simulink model "cw7_3_3"  (R2019a)
settings: Solver=VariableStepAuto  StartTime=0.0  StopTime=50  RelTol=1e-10  EnableMultiTasking=on
values from neighbouring files (symbols this model uses):
  k1 = 2    [SchematyBlokowe.m]    (also in TIPS_Lab_6_Zad_Dom.m = 0:N1-1)
  k2 = 2    [SchematyBlokowe.m]    (also in TIPS_Lab_6_Zad_Dom.m = 0:N2-1)
  kp = 5    [AutomatykaCw5.m]    (also in SchematyBlokowe.m = 2)
  kp1 = 0.3125    [SchematyBlokowe.m]
  kp2 = 0.2    [SchematyBlokowe.m]
  kp3 = 10    [SchematyBlokowe.m]
  T11 = 4    [SchematyBlokowe.m]
  T12 = 5    [SchematyBlokowe.m]
  T21 = 5    [SchematyBlokowe.m]
  T22 = 5    [SchematyBlokowe.m]
  Ti = 1    [SchematyBlokowe.m]
  Ti1 = 5    [SchematyBlokowe.m]
  Ti2 = 4    [SchematyBlokowe.m]
  Ti3 = 30    [SchematyBlokowe.m]
libraries: simulink x1
settings Model: Creator=Pawel  LastModifiedBy=ASUS_PEPE
settings DataIOCC: LimitDataPoints=on  ReturnWorkspaceOutputs=off
settings OptimizationCC: LifeSpan=inf
settings DebuggingCC: AllowSymbolicDim=off  SFUnexpectedBacktrackingDiag=warning  SFNoUnconditionalDefaultTransitionDiag=warning  SFExecutionAtInitializationDiag=none  ArithmeticOperatorsInVariantConditions=warning
settings ModelReferenceCC: PropagateSignalLabelsOutOfModel=off
settings SFSimCC: SimUseLocalCustomCode=off
settings RTWCC: RTWUseLocalCustomCode=off
settings CodeAppCC: StateflowObjectComments=on
settings GRTTargetCC: TargetLangStandard=C89/C90 (ANSI)
settings ConfigComp: CovMetricSettings=dw  CovHtmlReporting=on  CovSaveCumulativeToWorkspaceVar=on  CovSaveSingleToWorkspaceVar=on  CovExternalEMLEnable=off

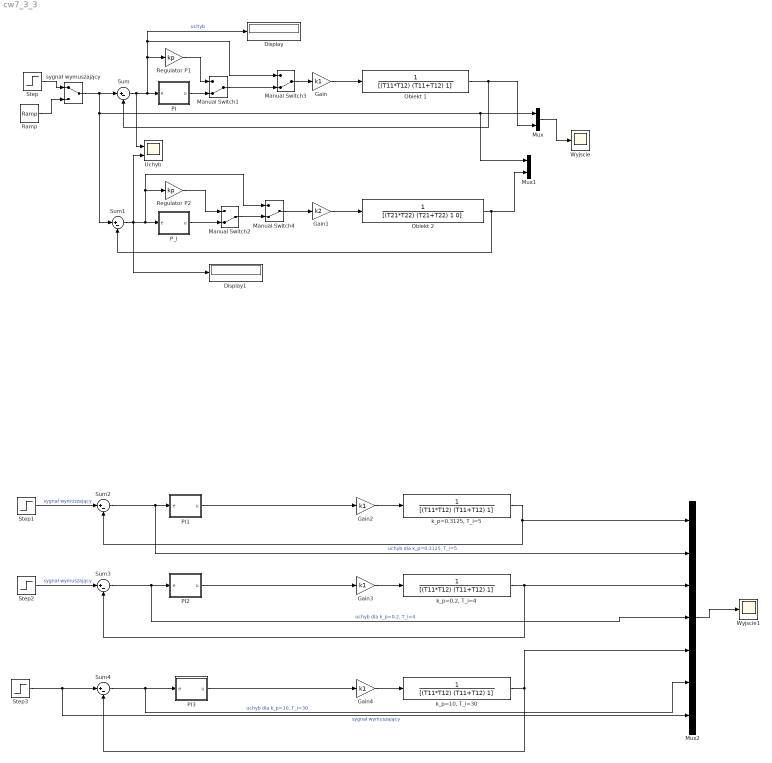
== system cw7_3_3 ==
  Display : Display
  Display1 : Display
  Gain{,2..4} (4 alike) : Gain  Gain=k1
  Gain1 : Gain  Gain=k2
  Manual Switch{1..4} (4 alike) : ManualSwitch  CurrentSetting=0
  Mux : Mux  Inputs=2
  Mux1 : Mux  Inputs=2
  Mux2 : Mux  Inputs=7
  Obiekt 1 : TransferFcn  Numerator=1  Denominator=[(T11*T12) (T11+T12) 1]
  Obiekt 2 : TransferFcn  Numerator=1  Denominator=[(T21*T22) (T21+T22) 1 0]
  PI : Subsystem
  "PI1 " : Subsystem
  PI2 : Subsystem
  PI3 : Subsystem
  P_I : Subsystem
  Ramp : simulink/Sources/Ramp  slope=1  start=0  InitialOutput=0
  Regulator P1 : Gain  Gain=kp
  Regulator P2 : Gain  Gain=kp
  Step : Step  SampleTime=0
  Step1 : Step  Before=1  SampleTime=0
  Step2 : Step  Before=1  SampleTime=0
  Step3 : Step  Before=1  SampleTime=0
  Sum{,1..4} (5 alike) : Sum  Inputs=|+-
  Uchyb : Scope  NumInputPorts=2
  Wyjscie : Scope
  Wyjscie1 : Scope
  "k_p=0.2, T_i=4" : TransferFcn  Numerator=1  Denominator=[(T11*T12) (T11+T12) 1]
  "k_p=0.3125, T_i=5" : TransferFcn  Numerator=1  Denominator=[(T11*T12) (T11+T12) 1]
  "k_p=10, T_i=30" : TransferFcn  Numerator=1  Denominator=[(T11*T12) (T11+T12) 1]
  sygnał wymuszający : ManualSwitch
  wires:
  Obiekt 1/1 -> Sum/2, Mux/2
  Sum/1 -> Manual Switch3/1, Display/1, Regulator P1/1, PI/1(e), Uchyb/1  "uchyb"
  Obiekt 2/1 -> Sum1/2, Mux1/2
  Sum1/1 -> Display1/1, Uchyb/2, Manual Switch4/1, Regulator P2/1, P_I/1(e)
  Gain/1 -> Obiekt 1/1
  Gain1/1 -> Obiekt 2/1
  sygnał wymuszający/1 -> Sum1/1, Mux1/1, Mux/1, Sum/1
  Step/1 -> sygnał wymuszający/1
  Ramp/1 -> sygnał wymuszający/2
  Manual Switch1/1 -> Manual Switch3/2
  PI/1(u) -> Manual Switch1/2
  Regulator P1/1 -> Manual Switch1/1
  Regulator P2/1 -> Manual Switch2/1
  P_I/1(u) -> Manual Switch2/2
  Manual Switch2/1 -> Manual Switch4/2
  Manual Switch3/1 -> Gain/1
  Manual Switch4/1 -> Gain1/1
  Mux/1 -> Wyjscie/1
  Step1/1 -> Sum2/1  "sygnał wymuszający"
  Gain2/1 -> "k_p=0.3125, T_i=5"/1
  "k_p=0.3125, T_i=5"/1 -> Sum2/2, Mux2/1
  PI3/1(u) -> Gain4/1
  PI2/1(u) -> Gain3/1
  "PI1 "/1(u) -> Gain2/1
  Sum2/1 -> Mux2/2, "PI1 "/1(e)  "uchyb dla k_p=0.3125, T_i=5"
  Gain4/1 -> "k_p=10, T_i=30"/1
  Gain3/1 -> "k_p=0.2, T_i=4"/1
  Sum3/1 -> Mux2/4, PI2/1(e)  "uchyb dla k_p=0.2, T_i=4"
  Step2/1 -> Sum3/1  "sygnał wymuszający"
  Sum4/1 -> Mux2/6, PI3/1(e)  "uchyb dla k_p=10, T_i=30"
  Step3/1 -> Mux2/7, Sum4/1  "sygnał wymuszający"
  "k_p=0.2, T_i=4"/1 -> Mux2/3, Sum3/2
  Mux2/1 -> Wyjscie1/1
  "k_p=10, T_i=30"/1 -> Mux2/5, Sum4/2

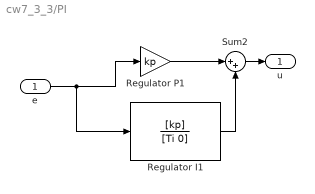
== system cw7_3_3/PI ==
  e : Inport
  Regulator I1 : TransferFcn  Numerator=[kp]  Denominator=[Ti 0]
  Regulator P1 : Gain  Gain=kp
  Sum2 : Sum  Inputs=|++
  u : Outport
  wires:
  Regulator I1/1 -> Sum2/2
  Sum2/1 -> u/1
  e/1 -> Regulator I1/1, Regulator P1/1
  Regulator P1/1 -> Sum2/1

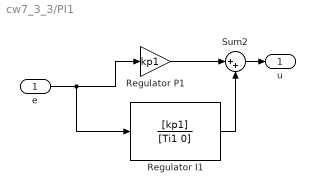
== system cw7_3_3/PI1  ==
  e : Inport
  Regulator I1 : TransferFcn  Numerator=[kp1]  Denominator=[Ti1 0]
  Regulator P1 : Gain  Gain=kp1
  Sum2 : Sum  Inputs=|++
  u : Outport
  wires:
  Regulator I1/1 -> Sum2/2
  Sum2/1 -> u/1
  e/1 -> Regulator I1/1, Regulator P1/1
  Regulator P1/1 -> Sum2/1

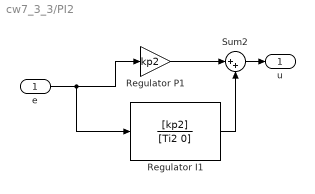
== system cw7_3_3/PI2 ==
  e : Inport
  Regulator I1 : TransferFcn  Numerator=[kp2]  Denominator=[Ti2 0]
  Regulator P1 : Gain  Gain=kp2
  Sum2 : Sum  Inputs=|++
  u : Outport
  wires:
  Regulator I1/1 -> Sum2/2
  Sum2/1 -> u/1
  e/1 -> Regulator I1/1, Regulator P1/1
  Regulator P1/1 -> Sum2/1

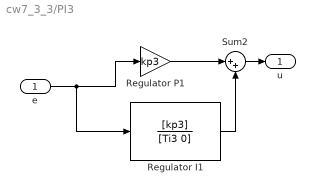
== system cw7_3_3/PI3 ==
  e : Inport
  Regulator I1 : TransferFcn  Numerator=[kp3]  Denominator=[Ti3 0]
  Regulator P1 : Gain  Gain=kp3
  Sum2 : Sum  Inputs=|++
  u : Outport
  wires:
  Regulator I1/1 -> Sum2/2
  Sum2/1 -> u/1
  e/1 -> Regulator I1/1, Regulator P1/1
  Regulator P1/1 -> Sum2/1

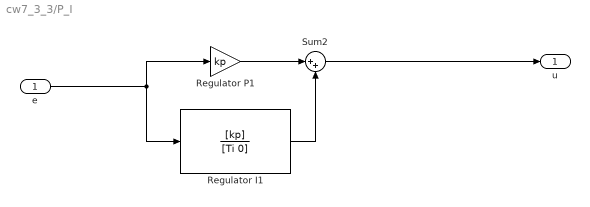
== system cw7_3_3/P_I ==
  e : Inport
  Regulator I1 : TransferFcn  Numerator=[kp]  Denominator=[Ti 0]
  Regulator P1 : Gain  Gain=kp
  Sum2 : Sum  Inputs=|++
  u : Outport
  wires:
  Regulator P1/1 -> Sum2/1
  e/1 -> Regulator P1/1, Regulator I1/1
  Sum2/1 -> u/1
  Regulator I1/1 -> Sum2/2
